simulink model "psbacdrive"  (Simulink 6.0)
settings: Solver=FixedStepDiscrete  SolverMode=SingleTasking  StartTime=0.0  StopTime=1.5  RelTol=1e-3
PreLoadFcn:
  | assignin('base','Ts',[2e-6])
InitFcn:
  | powericon('psbinitsys',bdroot);
undefined symbols (not defined in the file or in its folder): DiscIntNeverNeededParam, Ts
libraries: powerlib2 x7
settings Model: Creator=lehuy  LastModifiedBy=batserve  ExtModeTrigMode=oneshot  ExtModeArmWhenConnect=off  ExtModeAutoUpdateStatusClock=off
settings DataIOCC: LimitDataPoints=off  SaveFinalState=on  SaveFormat=StructureWithTime  SaveOutput=off  SaveTime=off  SignalLoggingName=sigsOut
settings OptimizationCC: BlockReduction=off
settings DebuggingCC: CheckExecutionContextPreStartOutputMsg=on  CheckExecutionContextRuntimeOutputMsg=on  SolverPrmCheckMsg=none  UnconnectedOutputMsg=none
settings HardwareCC: TargetUnknown=on
settings RTWCC: TemplateMakefile=grt_vc.tmf

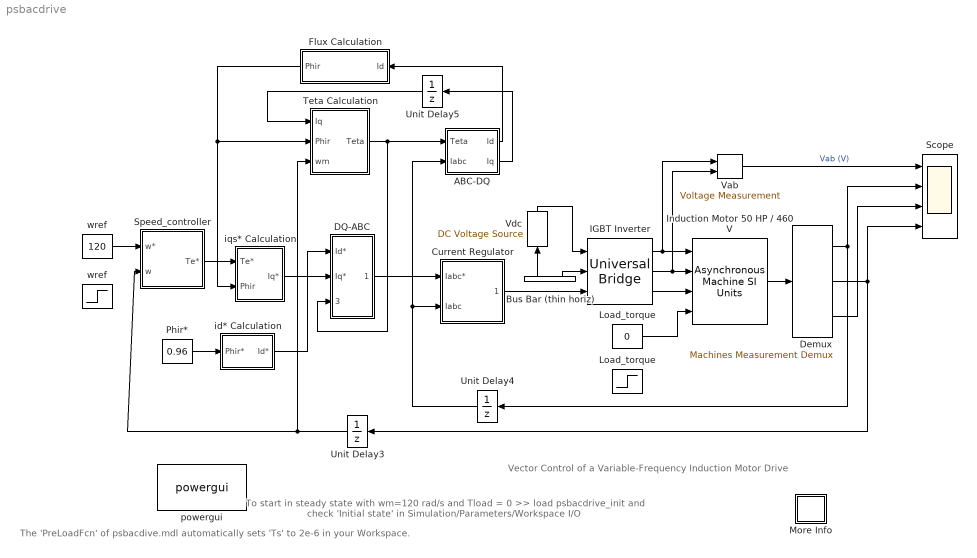
== system psbacdrive ==
  note: The 'PreLoadFcn' of psbacdive.mdl
      | automatically sets 'Ts' to 2e-6 in your Workspace.
  note: To start in steady state with wm=120 rad/s and Tload = 0
      | >> load psbacdrive_init
      | and check 'Initial state' in Simulation/Parameters/Workspace I/O
  note: Vector Control of a Variable-Frequency Induction Motor Drive
  ABC-DQ : Subsystem
  Bus Bar (thin horiz) : powerlib2/Connectors/Bus Bar (thin horiz)  Tag=PoWeRsYsTeMbLoCk  Orientation=up  input=0  output=2  PSBOutputType=111111111111111111111111111111111111111111111111111111111111111111111111111111111111
  Current Regulator : Subsystem  mask(Regulateur de courant a hysteresis){h=20}
      mask prompts: h "Hysteresis band (A)"
  DQ-ABC : Subsystem
  Demux : powerlib2/Machines/Machines Measurement Demux  machType=Asynchronous  ssm1=on  ssm2=on  ssm3=on  ssm4=on  ssm5=on  ssm6=on  sm1=on  sm2=on  sm3=on  sm4=on  sm5=on  sm6=on  sm7=on  sm8=on  sm9=on  sm10=on  sm11=on  sm115=off  sm12=off  sm13=off  sm14=off  asm1=off  asm2=off  asm3=off  asm4=off  asm5=on  asm6=off  asm7=off  asm8=off  asm9=on  asm10=on  asm11=off  pmsm1=on  pmsm2=on  pmsm3=on  pmsm4=on  pmsm5=on  pmsm6=on  lastType=3
  Flux Calculation : Subsystem  Orientation=left  mask(Flux Calcultation){}
      mask init:
      | NF=0.44572610323020e-6;
      | DF=[1 -0.99998715486734];
      mask Display: disp('Flux\nCalc.')
  IGBT Inverter : powerlib2/Power Electronics/Universal Bridge  Tag=PoWeRsYsTeMbLoCk  arms=3  confi=ABC as output terminals  injcc=1000  cf=inf  device=IGBT / Diodes  Ron=1e-3  Lon=0  VFs="[  0.8  0.8  ]"  Vf=.8  gtoparameters=[ 1e-6 , 1e-6 ]  igbtparameters=[ 1e-6 , 2e-6 ]  mesure=None  PSBOutputType=111
  Induction Motor 50 HP / 460 V : powerlib2/Machines/Asynchronous Machine SI Units  Tag=PoWeRsYsTeMbLoCk  rotType=Squirrel-cage  ctrl=Stationary  x1=[ 50*746, 460, 60 ]  x2=[ 0.087 0.8e-3 ]  x3="[ 0.228  0.8e-3 ]"  x4=34.7e-3  x5="[1.662  0.1 2 ]"  x6="[ 1, 0 ,  0 , 0 , 0 , 0 , 0 , 0 ]"  PSBOutputType=1110  iounits=1  LoadFlowParameters=0
  Load_torque : Step  Time=2  After=200  SampleTime=0
  "Load_torque " : Constant  Value=0
  More Info : Subsystem
      mask Display: disp('?')
  Phir* : Constant  Value=0.96
  Scope : Scope  NumInputPorts=4
      settings: TimeRange=0.03  YMin=-1000~-500~0~0  YMax=1000~500~400~6  Decimation=20  SampleTime=5e-6
  Speed_controller : Subsystem  mask(PI controller){Kp=13, Ki=26, Tlim=300, Ts=2e-6}
      mask prompts: Kp "Proportional gain (Kp)"; Ki "Integral gain (Ki)"; Tlim "Torque limit (N.m)"; Ts "Sampling time (s)"
      mask help: Proportional-Integral Speed Controller
      mask Display: plot(0,0,100,100,[35,35,65],[70,30,30],[35,65],[45,60])
  Teta Calculation : Subsystem
  Unit Delay3 : UnitDelay  Orientation=left  SampleTime=Ts
  Unit Delay4 : UnitDelay  Orientation=left  SampleTime=Ts
  Unit Delay5 : UnitDelay  Orientation=left  SampleTime=Ts
  Vab : powerlib2/Measurements/Voltage Measurement  Tag=PoWeRsYsTeMmEaSuReMeNt  PhasorSimulation=off  OutputType=Magnitude  PSBOutputType=0  PSBequivalent=0
  Vdc : powerlib2/Electrical Sources/DC Voltage Source  Tag=PoWeRsYsTeMbLoCk  Description=source block  Orientation=up  V=780  mesure=None  PSBOutputType=1
  id* Calculation : Subsystem
  iqs* Calculation : Subsystem
  powergui : powerlib2/powergui  Frange=[0:2:500]  Ylog=off  Xlog=on  save=off  variable=ZData  ZoomFFT=on  StartTime=0.0  cycles=1  DisplayStyle=off  fundamental=60  FreqAxis=off  MaxFrequency=1000  frequencyindice=1  frequencyindicesteady=1  RmsSteady=1  display=off  Ts=2e-6  methode=off  frequency=60  echomessages=off
  wref : Step  Time=0.4  Before=120  After=160  SampleTime=0
  "wref " : Constant  Value=120
  wires:
  DQ-ABC/1(Iabc*) -> Current Regulator/1(Iabc*)
  Speed_controller/1(Te*) -> iqs* Calculation/1(Te*)
  Phir*/1 -> id* Calculation/1(Phir*)
  ABC-DQ/1(Id) -> Flux Calculation/1(Id)
  Unit Delay4/1 -> Current Regulator/2(Iabc), ABC-DQ/2(Iabc)
  Teta Calculation/1(Teta) -> ABC-DQ/1(Teta), DQ-ABC/3(Teta)
  iqs* Calculation/1(Iq*) -> DQ-ABC/2(Iq*)
  id* Calculation/1(Id*) -> DQ-ABC/1(Id*)
  Flux Calculation/1(Phir) -> Teta Calculation/2(Phir), iqs* Calculation/2(Phir)
  Induction Motor 50 HP / 460 V/1 -> Demux/1
  Bus Bar (thin horiz)/1 -> Vdc/1
  Bus Bar (thin horiz)/2 -> IGBT Inverter/2
  Vdc/1 -> IGBT Inverter/1
  Current Regulator/1(Pulses) -> IGBT Inverter/3
  Vab/1 -> Scope/1  "Vab (V)"
  Demux/3 -> Scope/3
  Demux/2 -> Scope/4, Unit Delay3/1
  IGBT Inverter/3 -> Induction Motor 50 HP / 460 V/3
  IGBT Inverter/1 -> Induction Motor 50 HP / 460 V/1, Vab/1
  IGBT Inverter/2 -> Induction Motor 50 HP / 460 V/2, Vab/2
  Demux/1 -> Unit Delay4/1, Scope/2
  Unit Delay3/1 -> Teta Calculation/3(wm), Speed_controller/2(w)
  ABC-DQ/2(Iq) -> Unit Delay5/1
  Unit Delay5/1 -> Teta Calculation/1(Iq)
  "wref "/1 -> Speed_controller/1(w*)
  "Load_torque "/1 -> Induction Motor 50 HP / 460 V/4

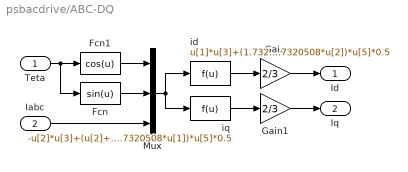
== system psbacdrive/ABC-DQ ==
  Teta : Inport  Port=1  LatchInput=off
  Iabc : Inport  Port=2  LatchInput=off
  Fcn : Fcn  Expr=sin(u)
  Fcn1 : Fcn  Expr=cos(u)
  Gain : Gain  Gain=2/3  SaturateOnIntegerOverflow=on
  Gain1 : Gain  Gain=2/3  SaturateOnIntegerOverflow=on
  Mux : Mux  Inputs=[1 1 3]
  id : Fcn  Expr=u[1]*u[3]+(1.7320508*u[2]-u[1])*u[4]*0.5+(-u[1]-1.7320508*u[2])*u[5]*0.5
  iq : Fcn  Expr=-u[2]*u[3]+(u[2]+1.7320508*u[1])*u[4]*0.5+(u[2]-1.7320508*u[1])*u[5]*0.5
  Id : Outport  InitialOutput=0
  Iq : Outport  Port=2  InitialOutput=0
  wires:
  Fcn/1 -> Mux/2
  Fcn1/1 -> Mux/1
  Teta/1 -> Fcn1/1, Fcn/1
  Mux/1 -> iq/1, id/1
  Iabc/1 -> Mux/3
  iq/1 -> Gain1/1
  id/1 -> Gain/1
  Gain/1 -> Id/1
  Gain1/1 -> Iq/1

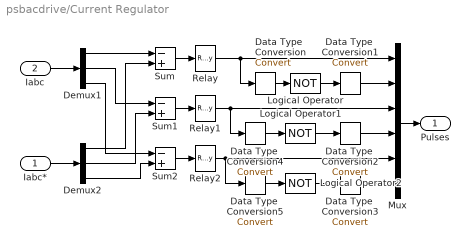
== system psbacdrive/Current Regulator ==
  Iabc* : Inport  Port=1  LatchInput=off
  Iabc : Inport  Port=2  LatchInput=off
  Data Type  Conversion : DataTypeConversion  OutDataTypeMode=boolean  SaturateOnIntegerOverflow=on  RndMeth=Zero
  Data Type  Conversion1 : DataTypeConversion  OutDataTypeMode=double  SaturateOnIntegerOverflow=on  RndMeth=Zero
  Data Type  Conversion2 : DataTypeConversion  OutDataTypeMode=double  SaturateOnIntegerOverflow=on  RndMeth=Zero
  Data Type  Conversion3 : DataTypeConversion  OutDataTypeMode=double  SaturateOnIntegerOverflow=on  RndMeth=Zero
  Data Type  Conversion4 : DataTypeConversion  OutDataTypeMode=boolean  SaturateOnIntegerOverflow=on  RndMeth=Zero
  Data Type  Conversion5 : DataTypeConversion  OutDataTypeMode=boolean  SaturateOnIntegerOverflow=on  RndMeth=Zero
  Demux1 : Demux  Outputs=3
  Demux2 : Demux  Outputs=3
  Logical Operator : Logic  Operator=NOT
  Logical Operator1 : Logic  Operator=NOT
  Logical Operator2 : Logic  Operator=NOT
  Mux : Mux  Inputs=6
  Relay : Relay  OnSwitchValue=h/2  OffSwitchValue=-h/2
  Relay1 : Relay  OnSwitchValue=h/2  OffSwitchValue=-h/2
  Relay2 : Relay  OnSwitchValue=h/2  OffSwitchValue=-h/2
  Sum : Sum  Inputs=-+  SaturateOnIntegerOverflow=on  InputSameDT=on
  Sum1 : Sum  Inputs=-+  SaturateOnIntegerOverflow=on  InputSameDT=on
  Sum2 : Sum  Inputs=-+  SaturateOnIntegerOverflow=on  InputSameDT=on
  Pulses : Outport  InitialOutput=0
  wires:
  Sum/1 -> Relay/1
  Sum1/1 -> Relay1/1
  Demux1/1 -> Sum/1
  Demux1/2 -> Sum1/1
  Mux/1 -> Pulses/1
  Iabc/1 -> Demux1/1
  Sum2/1 -> Relay2/1
  Demux1/3 -> Sum2/1
  Demux2/3 -> Sum2/2
  Demux2/2 -> Sum1/2
  Demux2/1 -> Sum/2
  Iabc*/1 -> Demux2/1
  Relay/1 -> Mux/1, Data Type  Conversion/1
  Relay1/1 -> Mux/3, Data Type  Conversion4/1
  Relay2/1 -> Mux/5, Data Type  Conversion5/1
  Data Type  Conversion/1 -> Logical Operator/1
  Logical Operator/1 -> Data Type  Conversion1/1
  Data Type  Conversion1/1 -> Mux/2
  Logical Operator1/1 -> Data Type  Conversion2/1
  Data Type  Conversion2/1 -> Mux/4
  Logical Operator2/1 -> Data Type  Conversion3/1
  Data Type  Conversion3/1 -> Mux/6
  Data Type  Conversion4/1 -> Logical Operator1/1
  Data Type  Conversion5/1 -> Logical Operator2/1

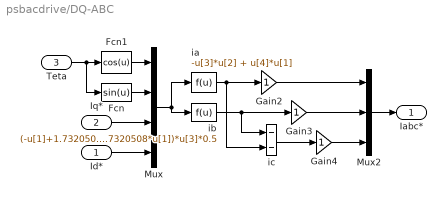
== system psbacdrive/DQ-ABC ==
  Id* : Inport  Port=1  LatchInput=off
  Iq* : Inport  Port=2  LatchInput=off
  Teta : Inport  Port=3  LatchInput=off
  Fcn : Fcn  Expr=sin(u)
  Fcn1 : Fcn  Expr=cos(u)
  Gain2 : Gain  SaturateOnIntegerOverflow=on
  Gain3 : Gain  SaturateOnIntegerOverflow=on
  Gain4 : Gain  SaturateOnIntegerOverflow=on
  Mux : Mux
  Mux2 : Mux  Inputs=3
  ia : Fcn  Expr=-u[3]*u[2] + u[4]*u[1]
  ib : Fcn  Expr=(-u[1]+1.7320508*u[2])*u[4]*0.5+(u[2]+1.7320508*u[1])*u[3]*0.5
  ic : Sum  Inputs=--  SaturateOnIntegerOverflow=on  InputSameDT=on
  Iabc* : Outport  InitialOutput=0
  wires:
  Fcn/1 -> Mux/2
  Fcn1/1 -> Mux/1
  Mux2/1 -> Iabc*/1
  Mux/1 -> ib/1, ia/1
  Teta/1 -> Fcn1/1, Fcn/1
  Iq*/1 -> Mux/3
  Id*/1 -> Mux/4
  Gain3/1 -> Mux2/2
  ic/1 -> Gain4/1
  Gain4/1 -> Mux2/3
  Gain2/1 -> Mux2/1
  ia/1 -> Gain2/1, ic/2
  ib/1 -> Gain3/1, ic/1

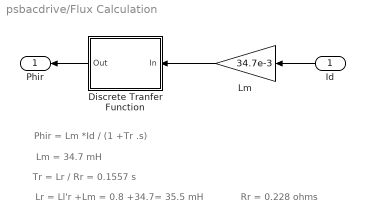
== system psbacdrive/Flux Calculation ==
  note: Phir = Lm *Id / (1 +Tr .s)
  note: Lm = 34.7 mH
  note: Lr = Ll'r +Lm = 0.8 +34.7= 35.5 mH
  note: Tr = Lr / Rr = 0.1557 s
  note: Rr = 0.228 ohms
  Id : Inport  Orientation=left  Port=1  LatchInput=off
  Discrete Tranfer Function : Subsystem  Orientation=left  mask(First Order Low Pass Filter (Discrete)){T=0.1557, Ts=2e-6}
      mask prompts: T "Time constant T (s) :"; Ts "Time step (s)"
      mask help: H(s)=1/(1+T.s)
      mask init:
      | X=[0 1 2 3 4];
      |  Y=[-2 -2 -3 -4 -4];
      |  str=sprintf('\nH=1/(1+T.s)\n T= %g s\n\n\n',T);
      | num=1;
      | den=[T 1];
      | 
      | % discrete transfer function
      | % descending powers of z
      | numd= Ts/T;
      | dend=[ 1  (Ts-T)/T];
      mask Display:
      | plot(X,Y);
      | disp(str);
  Lm : Gain  Orientation=left  Gain=34.7e-3  SaturateOnIntegerOverflow=on
  Phir : Outport  Orientation=left
  wires:
  Discrete Tranfer Function/1(Out) -> Phir/1
  Id/1 -> Lm/1
  Lm/1 -> Discrete Tranfer Function/1(In)

== system psbacdrive/More Info ==
  note: Start the simulation. Observe the motor current, voltage, speed, and torque during the starting on the scope.
      |
      | At the end of the simulation time (1.5 s), the system has attained its steady-state. The final state
      | vector can be saved by previously  selecting 'Workspace I/O/Save to workspace/Final state' in
      | Simulation/Parameters window.  Once the simultion is finished save the xFinal variable into xInitial.
      |
      | Note : The initial conditions state vector xInitial to start with wm = 120 rad/s and Te = 0  is stored in the
      | psbacdrive_init.mat file.
      |
      | Replace the constant wref and TL blocks by the two Simulink step functions with different starting times.
      | (Refence speed wref changed from 120 to 160 rad/s at t = 0.4 s and load torque changed from 0 to 200 N.m at t = 2s)
      | Select  'Workspace I/O/Load from workspace/Initial state' in Simulation parameters window to load the steady-state
      | vector xInitial.  Restart the simulation and  observe the drive response to successive changes in speed reference
      | and load torque.
  note: The induction motor is fed by a current-controlled PWM inverter which is built using a Universal Bridge block.
      | The motor drives a mechanical load characterized by inertia J, friction coeficient B, and load torque TL .
      | The speed control loop uses a proportional-integral controller to produce the quadrature-axis current reference
      | iq* which controls the motor torque.  The motor flux is controlled by the direct-axis current reference id*.
      | Block DQ-ABC is used to convert id* and iq* into current references ia*, ib*, and ic* for the current regulator.
      | Current and Voltage Measurement blocks provide signals for visualization purpose.
      | Motor current, speed, and torque signals are available at the output of the 'Asynchronous Machine' block.
  note: Demonstration
  note: Circuit Description
  note: Case study : Variable-Frequency Induction Motor Drive
  note: Notes
  note: 1) The system (control and power sytem) has been discretized with a 2 us time step.
  note: 2) In order to reduce the number of points stored in the scope memory, a decimation factor of 20 is used.
  note: H. Le-Huy (Universite Laval, Quebec)

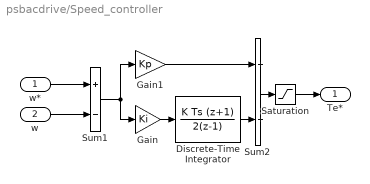
== system psbacdrive/Speed_controller ==
  w* : Inport  Port=1  LatchInput=off
  w : Inport  Port=2  LatchInput=off
  Discrete-Time Integrator : DiscreteIntegrator  IntegratorMethod=Integration: Trapezoidal  SampleTime=Ts  LimitOutput=on  UpperSaturationLimit=Tlim  LowerSaturationLimit=-Tlim  ICPrevOutput=DiscIntNeverNeededParam  ICPrevScaledInput=DiscIntNeverNeededParam
  Gain : Gain  Gain=Ki  SaturateOnIntegerOverflow=on
  Gain1 : Gain  Gain=Kp  SaturateOnIntegerOverflow=on
  Saturation : Saturate  UpperLimit=Tlim  LowerLimit=-Tlim
  Sum1 : Sum  Inputs=+-  SaturateOnIntegerOverflow=on  InputSameDT=on
  Sum2 : Sum  SaturateOnIntegerOverflow=on  InputSameDT=on
  Te* : Outport  InitialOutput=0
  wires:
  Gain1/1 -> Sum2/1
  Gain/1 -> Discrete-Time Integrator/1
  Sum1/1 -> Gain/1, Gain1/1
  Discrete-Time Integrator/1 -> Sum2/2
  Sum2/1 -> Saturation/1
  Saturation/1 -> Te*/1
  w/1 -> Sum1/2
  w*/1 -> Sum1/1

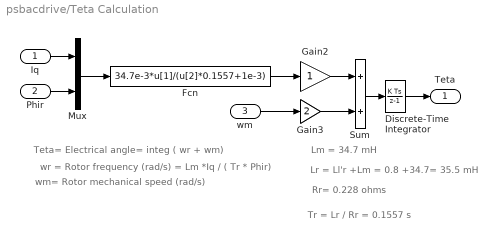
== system psbacdrive/Teta Calculation ==
  note: Teta= Electrical angle= integ ( wr + wm)
  note: wr = Rotor frequency (rad/s) = Lm *Iq / ( Tr * Phir)
  note: Lm = 34.7 mH
  note: Rr= 0.228 ohms
  note: Lr = Ll'r +Lm = 0.8 +34.7= 35.5 mH
  note: wm= Rotor mechanical speed (rad/s)
  note: Tr = Lr / Rr = 0.1557 s
  Iq : Inport  Port=1  LatchInput=off
  Phir : Inport  Port=2  LatchInput=off
  wm : Inport  Port=3  LatchInput=off
  Discrete-Time Integrator : DiscreteIntegrator  SampleTime=Ts  ICPrevOutput=DiscIntNeverNeededParam  ICPrevScaledInput=DiscIntNeverNeededParam
  Fcn : Fcn  Expr=34.7e-3*u[1]/(u[2]*0.1557+1e-3)
  Gain2 : Gain  SaturateOnIntegerOverflow=on
  Gain3 : Gain  Gain=2  SaturateOnIntegerOverflow=on
  Mux : Mux  Inputs=2
  Sum : Sum  SaturateOnIntegerOverflow=on  InputSameDT=on
  Teta : Outport  InitialOutput=0
  wires:
  Discrete-Time Integrator/1 -> Teta/1
  Sum/1 -> Discrete-Time Integrator/1
  Gain3/1 -> Sum/2
  Gain2/1 -> Sum/1
  wm/1 -> Gain3/1
  Fcn/1 -> Gain2/1
  Phir/1 -> Mux/2
  Iq/1 -> Mux/1
  Mux/1 -> Fcn/1

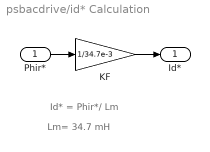
== system psbacdrive/id* Calculation ==
  note: Id* = Phir*/ Lm
  note: Lm= 34.7 mH
  Phir* : Inport  Port=1  LatchInput=off
  KF : Gain  Gain=1/34.7e-3  SaturateOnIntegerOverflow=on
  Id* : Outport
  wires:
  KF/1 -> Id*/1
  Phir*/1 -> KF/1

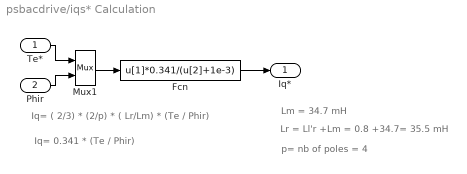
== system psbacdrive/iqs* Calculation ==
  note: Iq= ( 2/3) * (2/p) * ( Lr/Lm) * (Te / Phir)
  note: Lm = 34.7 mH
  note: Lr = Ll'r +Lm = 0.8 +34.7= 35.5 mH
  note: p= nb of poles = 4
  note: Iq= 0.341 * (Te / Phir)
  Te* : Inport  Port=1  LatchInput=off
  Phir : Inport  Port=2  LatchInput=off
  Fcn : Fcn  Expr=u[1]*0.341/(u[2]+1e-3)
  Mux1 : Mux  Inputs=2
  Iq* : Outport  InitialOutput=0
  wires:
  Phir/1 -> Mux1/2
  Fcn/1 -> Iq*/1
  Te*/1 -> Mux1/1
  Mux1/1 -> Fcn/1

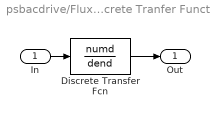
== system psbacdrive/Flux Calculation/Discrete Tranfer Function ==
  In : Inport  Port=1  LatchInput=off
  Discrete Transfer Fcn : DiscreteTransferFcn  Numerator=numd  Denominator=dend  SampleTime=Ts
  Out : Outport  InitialOutput=0
  wires:
  Discrete Transfer Fcn/1 -> Out/1
  In/1 -> Discrete Transfer Fcn/1
